simulink model "DC_MOTOR"  (R2018a)
settings: Solver=VariableStepAuto  StartTime=0.0  StopTime=27.2  RelTol=1e-3
model workspace (MAT data in the model file):
  B = 7.85992811423e-18
  J = 8.21678028349e-05
  K = 0.0136116359456
  L = 0.0010753661242
  R = 0.6
libraries: simulink_extras x2
settings Model: Creator=Hazem Elwakeel  LastModifiedBy=Hazem Elwakeel

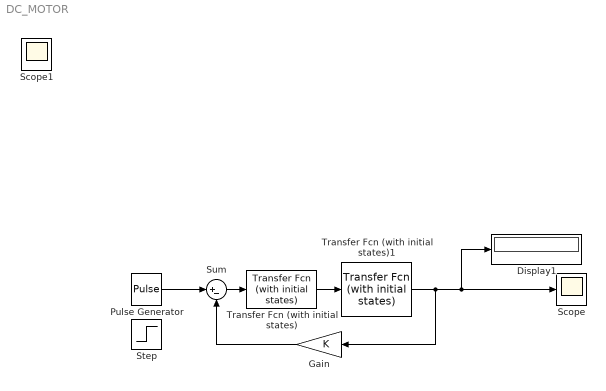
== system DC_MOTOR ==
  Display1 : Display
  Gain : Gain  Gain=K
  Pulse Generator : DiscretePulseGenerator  PulseType=Time based  Amplitude=12.08  Period=10  PulseWidth=50
  Scope : Scope
  Step : Step  Time=0  After=11  SampleTime=0
  Sum : Sum  Inputs=|+-
  Transfer Fcn (with initial states) : simulink_extras/Additional Linear/Transfer Fcn (with initial states)  N=[K]  D="[J  B]"  X0=.5
  Transfer Fcn (with initial states)1 : simulink_extras/Additional Linear/Transfer Fcn (with initial states)  N=[1]  D="[L  R]"  X0=.5
  Scope1 : Scope
  wires:
  Transfer Fcn (with initial states)/1 -> Transfer Fcn (with initial states)1/1
  Sum/1 -> Transfer Fcn (with initial states)/1
  Gain/1 -> Sum/2
  Transfer Fcn (with initial states)1/1 -> Gain/1, Display1/1, Scope/1
  Pulse Generator/1 -> Sum/1
